simulink model "campus"  (Simulink 7.9)
settings: Solver=FixedStepDiscrete  StartTime=0.0  StopTime=1*24*60*60  FixedStep=15*60  RelTol=1e-3
libraries: mlepLibrary x2
settings Model: Creator=willyg  LastModifiedBy=willyg

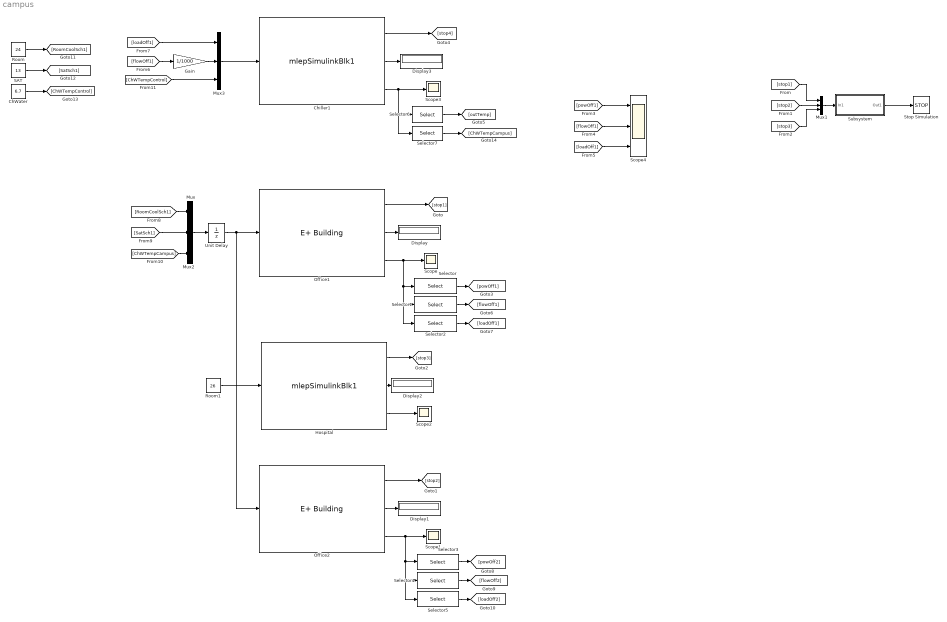
== system campus ==
  ChWater : Constant  Value=6.7
  Chiller1 : M-S-Function  AncestorBlock=mlepLibrary/E+ Building  FunctionName=mlepSimulinkBlk1  Parameters=progname, modelfile, weatherfile, workdir, timeout, port, host, bcvtbdir, deltaT, noutputd  mask(EnergyPlus Cosimulation){progname='runenergyplus', modelfile='/Users/willyg/Documents/Git/mlep_v2.0/CampusSimulation/Models/Chiller1/LargeChiller', weatherfile='USA_IL_Chicago-OHare.Intl.AP.725300_TMY3', workdir='/Users/willyg/Documents/Git/mlep_v2.0/CampusSimulation/Models/Chiller1', timeout=40000, port=0, host='', bcvtbdir='', deltaT=900, noutputd=2}
      mask prompts: progname "E+ Executable Path"; modelfile "IDF File (without extension)"; weatherfile "Weather Profile"; workdir "Working Directory"; timeout "Timeout (in milliseconds)"; port "Socket Port (0 = any available)"; host "Socket Host ('' = local host)"; bcvtbdir "BCVTB Directory"; deltaT "Time Step (in seconds)"; noutputd "Number of Real Outputs"
      mask help: This block implements cosimulation with EnergyPlus by allowing Simulink to exchange input and output data with it. Currently, EnergyPlus only supports real data.
      mask Help:
      | Simulate a building model using EnergyPlus
      | 
      | <h2>Description</h2>
      | This block implements <a href="http://apps1.eere.energy.gov/buildings/energyplus/">EnergyPlus</a> cosimulation by allowing Simulink to exchange input and output data with EnergyPlus at each time step.
      | 
      | When a simulation starts, this block starts EnergyPlus in parallel. During simulation, EnergyPlus exchanges data with Simulink using the <a href="http://simulationresearch.lbl.gov/bcvtb">Building Controls Virtual Test Bed</a> (BCVTB) interface via <a href="http://mlab.seas.upenn.edu/mlep/">MLE+</a>.
      | 
      | Detailed information about the interface is available in the MLE+ manual.
      | 
      | <h2>Requirements</h2>
      | Requires <a href="http://apps1.eere.energy.gov/buildings/energyplus/">EnergyPlus</a> and <a href="http://mlab.seas.upenn.edu/mlep/">MLE+</a>.
      | 
      | <h2>Input</h2>
      | Block input <b>real</b> is a real vector of EnergyPlus inputs corresponding to the inputs listed in the BCVTB config file <code>variables.cfg</code> (in order).
      | 
      | <h2>Output</h2>
      | The block outputs are, in order:
      | <dl>
      |   <dt><b>flag</b></dt><dd>Status flag for EnergyPlus: 0 if OK, non-zero for error</dd>
      |   <dt><b>time</b></dt><dd>Current simulation time of EnergyPlus (s)</dd>
      |   <dt><b>real</b></dt><dd>Real vector of EnergyPlus outputs corresponding to the outputs listed in the BCVTB config file <code>variables.cfg</code> (in order).</dd>
      | </dl>
      | 
      | <h2>Parameters</h2>
      | The block mask provides inputs for all required MLE+ configuration parameters:
      | <dl>
      |   <dt><b>E+ Executable Path</b></dt><dd>Specify the location of the EnergyPlus executable</dd>
      |   <dt><b>IDF File</b></dt><dd>Specify the EnergyPlus Input Description File (IDF), without extension</dd>
      |   <dt><b>Weather Profile</b></dt><dd>Specify the name of the EnergyPlus weather profile file to use for the model</dd>
      |   <dt><b>Working Directory</b></dt><dd>Specify the EnergyPlus working directory</dd>
      |   <dt><b>Timeout</b></dt><dd>Time delay (ms) before communication between MLE+ and EnergyPlus times out.</dd>
      |   <dt><b>Socket Port</b></dt><dd>Specify the port to use for communicating with EnergyPlus; enter <code>0</code> to use MLE+ default settings.</dd>
      |   <dt><b>Socket Host</b></dt><dd>Specifiy the IP address of the host where EnergyPlus runs; enter <code>''</code> to use localhost (the local computer).</dd>
      |   <dt><b>BCVTB Directory</b></dt><dd>Specify the directory where the BCVTB files reside; enter <code>''</code> to use MLE+ default settings.</dd>
      |   <dt><b>Time Step</b></dt><dd>Enter the EnergyPlus time step (s). This need not be the same as the Simulink time step.</dd>
      |   <dt><b>Number of Real Outputs</b></dt><dd>Specify the number of real outputs from EnergyPlus. This number should match the number of output variables in <code>variables.cfg</code>.</dd>
      | </dl>
      | 
      | All string inputs in the block mask must be passed either as MATLAB strings (that is, surrounded by single quotes <code>'</code>) or as MATLAB expressions which evaluate to strings (for example, <code>[pwd '/somedir']</code>).
      | 
      | <h2>Comments</h2>
      | <ol>
      |   <li>The BCVTB config file <code>variables.cfg</code> must be in the EnergyPlus working directory specified in the block mask.</li>
      |   <li>For fixed time step simulation in Simulink, the EnergyPlus time step should be an exact multiple of the Simulink time step.</li>
      |   <li>For details regarding the implementation of MLE+ and the meaning of the parameters, see the MLE+ <a href="http://mlab.seas.upenn.edu/mlep/">documentation</a>.</li>
      | </ol>
      | 
      | <h2>References</h2>
      | <ol>
      |   <li>W. Bernal, M. Behl, T. X. Nghiem, and R. Mangharam, "MLE+: A Tool for Integrated Design and Deployment of Energy Efficient Building Controls," 4th ACM Workshop On Embedded Sensing Systems For Energy-Efficiency In Buildings, (BuildSys '12), Toronto, Canada, 2012. Available: <a href="http://repository.upenn.edu/mlab_papers/51/">http://repository.upenn.edu/mlab_papers/51/</a></li>
      | </ol>
      mask Display:
      | image(imread('chiller_plant.jpg'))
      | disp('E+\nCosimulation');
      | 
      | % Inputs
      | port_label('input', 1, 'real');
      | 
      | % Outputs
      | port_label('output', 1, 'flag');
      | port_label('output', 2, 'time');
      | port_label('output', 3, 'real');
  Display{,1..3} (4 alike) : Display
  Gain : Gain  Gain=1/1000
  Hospital : M-S-Function  AncestorBlock=mlepLibrary/E+ Building  FunctionName=mlepSimulinkBlk1  Parameters=progname, modelfile, weatherfile, workdir, timeout, port, host, bcvtbdir, deltaT, noutputd  mask(EnergyPlus Cosimulation){progname='runenergyplus', modelfile='/Users/willyg/Documents/Git/mlep_v2.0/CampusSimulation/Models/Hospital1/Hospital', weatherfile='USA_IL_Chicago-OHare.Intl.AP.725300_TMY3', workdir='/Users/willyg/Documents/Git/mlep_v2.0/CampusSimulation/Models/Hospital1', timeout=40000, port=0, host='', bcvtbdir='', deltaT=900, noutputd=2}
      mask prompts: progname "E+ Executable Path"; modelfile "IDF File (without extension)"; weatherfile "Weather Profile"; workdir "Working Directory"; timeout "Timeout (in milliseconds)"; port "Socket Port (0 = any available)"; host "Socket Host ('' = local host)"; bcvtbdir "BCVTB Directory"; deltaT "Time Step (in seconds)"; noutputd "Number of Real Outputs"
      mask help: This block implements cosimulation with EnergyPlus by allowing Simulink to exchange input and output data with it. Currently, EnergyPlus only supports real data.
      mask Help:
      | Simulate a building model using EnergyPlus
      | 
      | <h2>Description</h2>
      | This block implements <a href="http://apps1.eere.energy.gov/buildings/energyplus/">EnergyPlus</a> cosimulation by allowing Simulink to exchange input and output data with EnergyPlus at each time step.
      | 
      | When a simulation starts, this block starts EnergyPlus in parallel. During simulation, EnergyPlus exchanges data with Simulink using the <a href="http://simulationresearch.lbl.gov/bcvtb">Building Controls Virtual Test Bed</a> (BCVTB) interface via <a href="http://mlab.seas.upenn.edu/mlep/">MLE+</a>.
      | 
      | Detailed information about the interface is available in the MLE+ manual.
      | 
      | <h2>Requirements</h2>
      | Requires <a href="http://apps1.eere.energy.gov/buildings/energyplus/">EnergyPlus</a> and <a href="http://mlab.seas.upenn.edu/mlep/">MLE+</a>.
      | 
      | <h2>Input</h2>
      | Block input <b>real</b> is a real vector of EnergyPlus inputs corresponding to the inputs listed in the BCVTB config file <code>variables.cfg</code> (in order).
      | 
      | <h2>Output</h2>
      | The block outputs are, in order:
      | <dl>
      |   <dt><b>flag</b></dt><dd>Status flag for EnergyPlus: 0 if OK, non-zero for error</dd>
      |   <dt><b>time</b></dt><dd>Current simulation time of EnergyPlus (s)</dd>
      |   <dt><b>real</b></dt><dd>Real vector of EnergyPlus outputs corresponding to the outputs listed in the BCVTB config file <code>variables.cfg</code> (in order).</dd>
      | </dl>
      | 
      | <h2>Parameters</h2>
      | The block mask provides inputs for all required MLE+ configuration parameters:
      | <dl>
      |   <dt><b>E+ Executable Path</b></dt><dd>Specify the location of the EnergyPlus executable</dd>
      |   <dt><b>IDF File</b></dt><dd>Specify the EnergyPlus Input Description File (IDF), without extension</dd>
      |   <dt><b>Weather Profile</b></dt><dd>Specify the name of the EnergyPlus weather profile file to use for the model</dd>
      |   <dt><b>Working Directory</b></dt><dd>Specify the EnergyPlus working directory</dd>
      |   <dt><b>Timeout</b></dt><dd>Time delay (ms) before communication between MLE+ and EnergyPlus times out.</dd>
      |   <dt><b>Socket Port</b></dt><dd>Specify the port to use for communicating with EnergyPlus; enter <code>0</code> to use MLE+ default settings.</dd>
      |   <dt><b>Socket Host</b></dt><dd>Specifiy the IP address of the host where EnergyPlus runs; enter <code>''</code> to use localhost (the local computer).</dd>
      |   <dt><b>BCVTB Directory</b></dt><dd>Specify the directory where the BCVTB files reside; enter <code>''</code> to use MLE+ default settings.</dd>
      |   <dt><b>Time Step</b></dt><dd>Enter the EnergyPlus time step (s). This need not be the same as the Simulink time step.</dd>
      |   <dt><b>Number of Real Outputs</b></dt><dd>Specify the number of real outputs from EnergyPlus. This number should match the number of output variables in <code>variables.cfg</code>.</dd>
      | </dl>
      | 
      | All string inputs in the block mask must be passed either as MATLAB strings (that is, surrounded by single quotes <code>'</code>) or as MATLAB expressions which evaluate to strings (for example, <code>[pwd '/somedir']</code>).
      | 
      | <h2>Comments</h2>
      | <ol>
      |   <li>The BCVTB config file <code>variables.cfg</code> must be in the EnergyPlus working directory specified in the block mask.</li>
      |   <li>For fixed time step simulation in Simulink, the EnergyPlus time step should be an exact multiple of the Simulink time step.</li>
      |   <li>For details regarding the implementation of MLE+ and the meaning of the parameters, see the MLE+ <a href="http://mlab.seas.upenn.edu/mlep/">documentation</a>.</li>
      | </ol>
      | 
      | <h2>References</h2>
      | <ol>
      |   <li>W. Bernal, M. Behl, T. X. Nghiem, and R. Mangharam, "MLE+: A Tool for Integrated Design and Deployment of Energy Efficient Building Controls," 4th ACM Workshop On Embedded Sensing Systems For Energy-Efficiency In Buildings, (BuildSys '12), Toronto, Canada, 2012. Available: <a href="http://repository.upenn.edu/mlab_papers/51/">http://repository.upenn.edu/mlab_papers/51/</a></li>
      | </ol>
      mask Display:
      | image(imread('building.png'))
      | disp('E+\nCosimulation');
      | 
      | % Inputs
      | port_label('input', 1, 'real');
      | 
      | % Outputs
      | port_label('output', 1, 'flag');
      | port_label('output', 2, 'time');
      | port_label('output', 3, 'real');
  Mux{,1..3} (4 alike) : Mux  Inputs=3
  Office1 : mlepLibrary/E+ Building  progname='runenergyplus'  modelfile='/Users/willyg/Documents/Git/mlep_v2.0/CampusSimulation/Models/Office1/LargeOffice'  weatherfile='USA_IL_Chicago-OHare.Intl.AP.725300_TMY3'  workdir='/Users/willyg/Documents/Git/mlep_v2.0/CampusSimulation/Models/Office1'  timeout=40000  port=0  host=''  bcvtbdir=''  deltaT=900  noutputd=6
  Office2 : mlepLibrary/E+ Building  progname='runenergyplus'  modelfile='/Users/willyg/Documents/Git/mlep_v2.0/CampusSimulation/Models/Office2/LargeOffice'  weatherfile='USA_IL_Chicago-OHare.Intl.AP.725300_TMY3'  workdir='/Users/willyg/Documents/Git/mlep_v2.0/CampusSimulation/Models/Office2'  timeout=40000  port=0  host=''  bcvtbdir=''  deltaT=900  noutputd=6
  Room : Constant  Value=24
  Room1 : Constant  Value=26
  SAT : Constant  Value=13
  Scope{,1..3} (4 alike) : Scope
      Scope settings: YMin=0  YMax=1.4e+09
      Scope1 settings: YMin=0  YMax=1.4e+09
      Scope2 settings: YMin=0  YMax=1.4e+09  SaveName=ScopeData2
      Scope3 settings: YMin=0  YMax=1.4e+09  SaveName=ScopeData3
  Scope4 : Scope  NumInputPorts=3
      settings: ShowLegends=on  YMin=0~-5~-5  YMax=1.4e+09~5~5  SaveName=ScopeData4
  Selector : Selector  InputPortWidth=6  IndexOptions=Index vector (dialog)  Indices=[2]  OutputSizes=1
  Selector1 : Selector  InputPortWidth=6  IndexOptions=Index vector (dialog)  Indices=[3]  OutputSizes=1
  Selector2 : Selector  InputPortWidth=6  IndexOptions=Index vector (dialog)  Indices=[4]  OutputSizes=1
  Selector3 : Selector  InputPortWidth=6  IndexOptions=Index vector (dialog)  Indices=[2]  OutputSizes=1
  Selector4 : Selector  InputPortWidth=6  IndexOptions=Index vector (dialog)  Indices=[3]  OutputSizes=1
  Selector5 : Selector  InputPortWidth=6  IndexOptions=Index vector (dialog)  Indices=[4]  OutputSizes=1
  Selector6 : Selector  InputPortWidth=2  IndexOptions=Index vector (dialog)  Indices=[1]  OutputSizes=1
  Selector7 : Selector  InputPortWidth=2  IndexOptions=Index vector (dialog)  Indices=[2]  OutputSizes=1
  Stop Simulation : Stop
  Subsystem : Subsystem
  Unit Delay : UnitDelay  SampleTime=-1
  wires:
  Office1/2 -> Display/1
  Office1/3 -> Scope/1, Selector/1, Selector1/1, Selector2/1
  Office2/1 -> [stop2]
  Office2/2 -> Display1/1
  Hospital/1 -> [stop3]
  Hospital/2 -> Display2/1
  Hospital/3 -> Scope2/1
  Room1/1 -> Hospital/1
  Office1/1 -> [stop1]
  [stop1] -> Mux1/1
  [stop2] -> Mux1/2
  [stop3] -> Mux1/3
  Mux1/1 -> Subsystem/1(In1)
  Subsystem/1(Out1) -> Stop Simulation/1
  Chiller1/2 -> Display3/1
  Chiller1/3 -> Scope3/1, Selector7/1, Selector6/1
  Chiller1/1 -> [stop4]
  Mux3/1 -> Chiller1/1
  Selector/1 -> [powOff1]
  Selector1/1 -> [flowOff1]
  Selector2/1 -> [loadOff1]
  [powOff1] -> Scope4/1
  [flowOff1] -> Scope4/2
  [loadOff1] -> Scope4/3
  [loadOff1] -> Mux3/1
  [flowOff1] -> Gain/1
  Gain/1 -> Mux3/2
  Office2/3 -> Scope1/1, Selector3/1, Selector4/1, Selector5/1
  Selector3/1 -> [powOff2]
  Selector4/1 -> [flowOff2]
  Selector5/1 -> [loadOff2]
  Mux/1 -> Unit Delay/1
  [RoomCoolSch1] -> Mux/1
  [SatSch1] -> Mux/2
  [ChWTempCampus] -> Mux/3
  Room/1 -> [RoomCoolSch1]
  SAT/1 -> [SatSch1]
  ChWater/1 -> [ChWTempControl]
  Selector6/1 -> [outTemp]
  Selector7/1 -> [ChWTempCampus]
  [ChWTempControl] -> Mux3/3
  Unit Delay/1 -> Office1/1, Office2/1

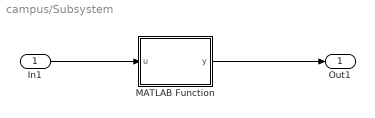
== system campus/Subsystem ==
  In1 : Inport
  MATLAB Function : MATLAB Function  TreatAsAtomicUnit=on
  Out1 : Outport
  wires:
  In1/1 -> MATLAB Function/1(u)
  MATLAB Function/1(y) -> Out1/1

== matlab function Subsystem/MATLAB Function ==
  data: u input double; y output double
function y = fcn(u)
%#codegen
% Number of Inputs
len = length(u);

% Check 
if sum(u==1) == len
    y = 1;
else
    y = 0;
end
